simulink model "Main_Model_CB_EN_UEEE23112"  (R2025b)
settings: Solver=ode23t  StartTime=0.0  StopTime=25  MaxStep=1e-5  RelTol=1e-3  AbsTol=1e-4
values from neighbouring files (symbols this model uses):
  Tsc = 5e-5    (= 5e-05)    [Model_Parameters_CB_EN_U4EEE23112.m]
undefined symbols (not defined in the file or in its folder): dspblkCoreblockFVToolHelper, gcbh
libraries: nesl_utility x31, fl_lib x20, ee_lib x12, sdl_lib x4, batteryecm_lib x1, eePmsmFieldOrientedControl x1
(part 3 of 3)

== stateflow chart Main_Model_CB_EN_UEEE23112/Brake and Control/Chart ==
  settings: executeAtInitialization=1
  state Normal_Operation
    state DRIVING
      en, du:
      speed_cmd_kmh = speed_kmh;
      pressure_cmd = 0;
    state REGEN
      en:
      pressure_cmd = 0;
      du:
      speed_cmd_kmh = max(0, speed_kmh - (brake_demand * 20));
      pressure_cmd = 0;
      ex:
      speed_cmd_kmh = speed_kmh;
    state BLEND_BRAKING
      en:
      pressure_cmd = 0;
      regen_gain = 0;
      du:
      % Cap gain at 1.0 to prevent runaway math at high speeds
      regen_gain = min(1, max(0, (speed_kmh - 3) / 7));
      speed_cmd_kmh = max(0, speed_kmh - (brake_demand * 20 * regen_gain));
      pressure_cmd = (1 - regen_gain) * brake_demand;
      ex:
      speed_cmd_kmh = speed_kmh;
      pressure_cmd = 0;
    state MECHANICAL_ONLY_BRAKING
      en, du:
      % Pass through speed to coast the motor
      speed_cmd_kmh = speed_kmh;
      pressure_cmd = brake_demand;
      ex:
      % Release the calipers before transitioning out
      pressure_cmd = 0;
    state Emergengy_regen
      en, du:
      % 1. Isolate the failed mechanical brakes
      pressure_cmd = 0;
      % 2. Force maximum regenerative braking
      % Setting the target speed to 0 forces the motor controller
      % to apply maximum negative torque to halt the vehicle.
      speed_cmd_kmh = 0;
      ex:
      % Sync the speed command back to actual speed if the fault clears
      speed_cmd_kmh = speed_kmh;
    (default) -> DRIVING
    DRIVING -> MECHANICAL_ONLY_BRAKING [order 2] : [brake_demand > 0.80 || SOC_pct >95]
    MECHANICAL_ONLY_BRAKING -> DRIVING [order 1] : [brake_demand < 0.02]
    BLEND_BRAKING -> DRIVING [order 2] : [brake_demand < 0.02]
    REGEN -> DRIVING [order 2] : [brake_demand < 0.02]
    DRIVING -> REGEN [order 1] : [brake_demand > 0.05 && speed_kmh > 5 && SOC_pct < 95]
    REGEN -> BLEND_BRAKING [order 1] : [brake_demand > 0.6 || speed_kmh < 10]
    BLEND_BRAKING -> MECHANICAL_ONLY_BRAKING [order 1] : [speed_kmh < 5 || SOC_pct >= 95 || brake_demand > 0.80]
    Emergengy_regen -> MECHANICAL_ONLY_BRAKING [order 2] : [Brake_fault==0 && brake_demand > 0.80]
    Emergengy_regen -> BLEND_BRAKING [order 1] : [Brake_fault==0]
    BLEND_BRAKING -> Emergengy_regen [order 3] : [Brake_fault==1]
    MECHANICAL_ONLY_BRAKING -> Emergengy_regen [order 2] : [Brake_fault==1]
  state Fault
    en, du:
    % Pass through speed to coast the motor
    speed_cmd_kmh = speed_kmh;
    pressure_cmd = 0.15;
    ex:
    % Release the calipers before transitioning out
    pressure_cmd = 0;
  (default) -> Normal_Operation
  Fault -> Normal_Operation : [Inveter_Fault==0 && Thermal_Fault==0]
  Normal_Operation -> Fault : [Inveter_Fault==1|| Thermal_Fault==1]
  data: brake_demand input; speed_kmh input; SOC_pct input; pressure_cmd output; regen_gain local; speed_cmd_kmh output; Thermal_Fault input; Inveter_Fault input; Brake_fault input
